simulink model "WPT_dc_source"  (R2022b)
settings: Solver=VariableStepAuto  StartTime=0.0  StopTime=10.0  RelTol=1e-3
libraries: spsMosfetLib x8, spsSeriesRLCBranchLib x6, spsVoltageMeasurementLib x6, spsDiodeLib x4, spsDCVoltageSourceLib x2, spsMutualInductanceLib x2, sps_lib x2
settings Model: Creator=SIDDHARTH  LastModifiedBy=SIDDHARTH

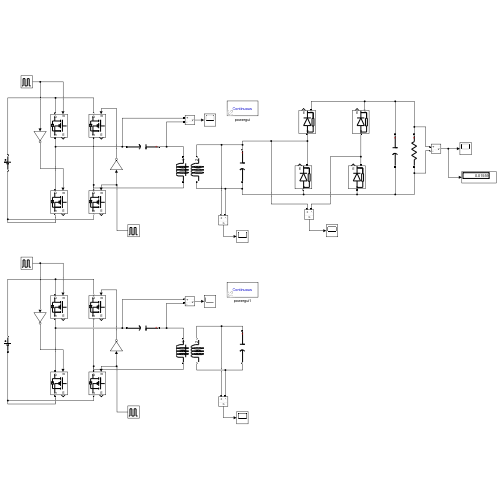
[thumbnail: Simulink's stored preview of the top-level diagram]
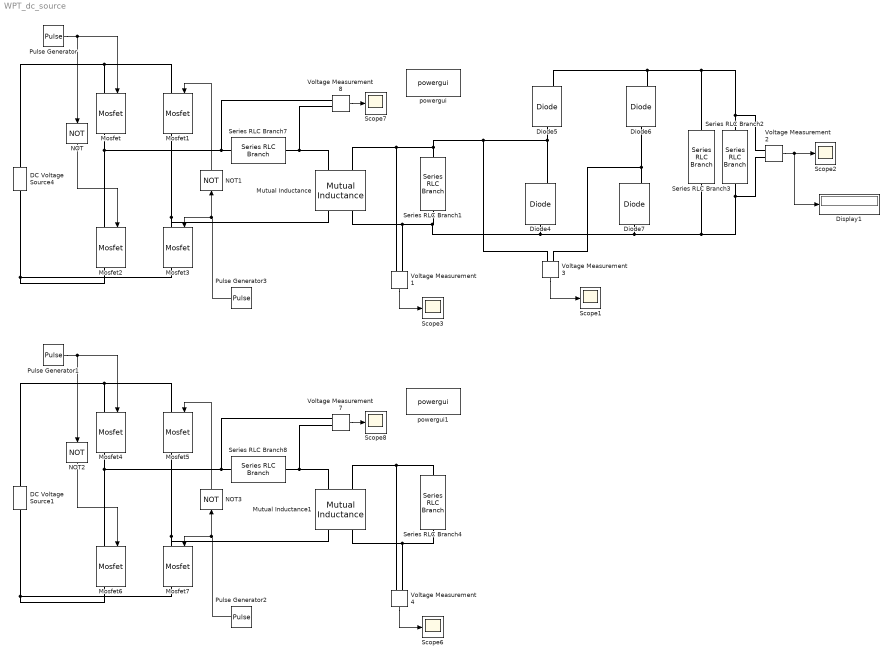
== system WPT_dc_source ==
  DC Voltage Source1 : spsDCVoltageSourceLib/DC Voltage Source  Amplitude=24  Measurements=None
  DC Voltage Source4 : spsDCVoltageSourceLib/DC Voltage Source  Amplitude=24  Measurements=None
  Diode4 : spsDiodeLib/Diode  Ron=0.001  Lon=0  Vf=0.7  IC=0  UseSnubber=0  Rs=500  Cs=250e-9  Measurements=on
  Diode5 : spsDiodeLib/Diode  Ron=0.001  Lon=0  Vf=0.8  IC=0  UseSnubber=0  Rs=500  Cs=250e-9  Measurements=on
  Diode6 : spsDiodeLib/Diode  Ron=0.001  Lon=0  Vf=0.7  IC=0  UseSnubber=0  Rs=500  Cs=250e-9  Measurements=on
  Diode7 : spsDiodeLib/Diode  Ron=0.001  Lon=0  Vf=0.7  IC=0  UseSnubber=0  Rs=500  Cs=250e-9  Measurements=on
  Display1 : Display
  Mosfet{,1..7} (8 alike) : spsMosfetLib/Mosfet  Ron=0.1  Lon=0  Rd=0.01  Vfd=0  IC=0  Rs=1e5  Cs=inf  Measurements=on
  Mutual Inductance : spsMutualInductanceLib/Mutual Inductance  LConnTagsString=a|b  RConnTagsString=A|B  TypeOfMutual=Two or three windings with equal mutual terms  NumberOfWindings=2  SelfImpedance1=[1e-2 1/(4*pi*pi*20000*(100e-6))]  SelfImpedance2=[1e-2 1/(4*pi*pi*20000*(100e-6))]  ThreeWindings=off  SelfImpedance3=[ 1.1 1.1e-03]  MutualImpedance=[0.9e-2 1.1207e-04]  InductanceMatrix="[1.0 0.9  0.9 ;  0.9 1.0  0.9;  0.9 0.9 1.0 ] * 1e-3"  ResistanceMatrix="[1.0 0.9  0.9 ;  0.9 1.0  0.9;  0.9 0.9 1.0 ]"  Measurements=Winding voltages
      settings: LibrarySourceBlock=sps_lib/Passives/Mutual Inductance
  Mutual Inductance1 : spsMutualInductanceLib/Mutual Inductance  LConnTagsString=a|b  RConnTagsString=A|B  TypeOfMutual=Two or three windings with equal mutual terms  NumberOfWindings=2  SelfImpedance1=[ 1.6054e-04 1/(4*pi*pi*20000*(100e-6))]  SelfImpedance2=[ 1.6054e-04 1/(4*pi*pi*20000*(100e-6))]  ThreeWindings=off  SelfImpedance3=[ 1.1 1.1e-03]  MutualImpedance=[ 1.6e-04 0.0099]  InductanceMatrix="[1.0 0.9  0.9 ;  0.9 1.0  0.9;  0.9 0.9 1.0 ] * 1e-3"  ResistanceMatrix="[1.0 0.9  0.9 ;  0.9 1.0  0.9;  0.9 0.9 1.0 ]"  Measurements=Winding voltages
      settings: LibrarySourceBlock=sps_lib/Passives/Mutual Inductance
  NOT{,1..3} (4 alike) : Logic  Operator=NOT  IconShape=distinctive  AllPortsSameDT=off  OutDataTypeStr=boolean
  Pulse Generator{,1..3} (4 alike) : DiscretePulseGenerator  PulseType=Time based  Period=1/20000  PulseWidth=75
  Scope{1..3,6..8} (6 alike) : Scope
  Series RLC Branch{1,4,7..8} (4 alike) : spsSeriesRLCBranchLib/Series RLC Branch  LConnTagsString=__new0  RConnTagsString=__new0  BranchType=C  Resistance=10  Inductance=1.02  SetiL0=off  InitialCurrent=0  Capacitance=100e-6  Setx0=off  InitialVoltage=0  Measurements=None
  Series RLC Branch2 : spsSeriesRLCBranchLib/Series RLC Branch  LConnTagsString=__new0  RConnTagsString=__new0  BranchType=R  Resistance=100000  Inductance=1e-3  SetiL0=off  InitialCurrent=0  Capacitance=1e-6  Setx0=off  InitialVoltage=0  Measurements=None
  Series RLC Branch3 : spsSeriesRLCBranchLib/Series RLC Branch  LConnTagsString=__new0  RConnTagsString=__new0  BranchType=C  Resistance=1  Inductance=1e-3  SetiL0=off  InitialCurrent=0  Capacitance=100e-6  Setx0=off  InitialVoltage=0  Measurements=Branch voltage
  Voltage Measurement{1..4,7..8} (6 alike) : spsVoltageMeasurementLib/Voltage Measurement  PhasorSimulation=off  OutputType=Complex  PSBequivalent=0
  powergui : sps_lib/powergui  Priority=1  SimulationMode=Continuous  SampleTime=50e-6  frequency=60  Iterations=50  frequencyindice=0  Pbase=100e6  ErrMax=1e-4  UnitsV=kV  UnitsW=MW  buscounter=0  FunctionMessages=off  echomessages=off  EnableUseOfTLC=off  CurrentSourceSwitches=off  DisableSnubberDevices=off  DisableRonSwitches=off  DisableVfSwitches=off  DisplayEquations=off  AutomaticDiscreteSolvers=off  SolverType=Tustin/Backward Euler (TBE)  Interpol=off  ExternalGateDelay=off  methode=off  Ts=100  x0status=blocks  SPID=on  SwTol=0  HookPort=off  NonlinearTolerance=1e-4  nMaxIteration=100  ContinueOnMaxIteration=off  RestoreLinks=warning  ResistiveCurrentMeasurement=off  Frange=[0:2:500]  Ylog=off  Xlog=on  ShowGrid=off  save=off  variable=ZData  structure=0  ZoomFFT=off  StartTime=0.0  cycles=1  DisplayStyle=1  fundamental=60  FreqAxis=off  MaxFrequency=1000  frequencyindicesteady=1  RmsSteady=1  display=off
  powergui1 : sps_lib/powergui  Priority=1  SimulationMode=Continuous  SampleTime=50e-6  frequency=60  Iterations=50  frequencyindice=0  Pbase=100e6  ErrMax=1e-4  UnitsV=kV  UnitsW=MW  buscounter=0  FunctionMessages=off  echomessages=off  EnableUseOfTLC=off  CurrentSourceSwitches=off  DisableSnubberDevices=off  DisableRonSwitches=off  DisableVfSwitches=off  DisplayEquations=off  AutomaticDiscreteSolvers=off  SolverType=Tustin/Backward Euler (TBE)  Interpol=off  ExternalGateDelay=off  methode=off  Ts=100  x0status=blocks  SPID=on  SwTol=0  HookPort=off  NonlinearTolerance=1e-4  nMaxIteration=100  ContinueOnMaxIteration=off  RestoreLinks=warning  ResistiveCurrentMeasurement=off  Frange=[0:2:500]  Ylog=off  Xlog=on  ShowGrid=off  save=off  variable=ZData  structure=0  ZoomFFT=off  StartTime=0.0  cycles=1  DisplayStyle=1  fundamental=60  FreqAxis=off  MaxFrequency=1000  frequencyindicesteady=1  RmsSteady=1  display=off
  wires:
  NOT/1 -> Mosfet2/1
  Pulse Generator3/1 -> NOT1/1, Mosfet3/1
  NOT1/1 -> Mosfet1/1
  Pulse Generator/1 -> Mosfet/1, NOT/1
  Voltage Measurement8/1 -> Scope7/1
  Voltage Measurement2/1 -> Display1/1, Scope2/1
  Voltage Measurement3/1 -> Scope1/1
  Voltage Measurement1/1 -> Scope3/1
  Pulse Generator2/1 -> NOT3/1, Mosfet7/1
  NOT2/1 -> Mosfet6/1
  NOT3/1 -> Mosfet5/1
  Voltage Measurement4/1 -> Scope6/1
  Pulse Generator1/1 -> Mosfet4/1, NOT2/1
  Voltage Measurement7/1 -> Scope8/1
  connections:
  Series RLC Branch7/LConn1 -- Mutual Inductance/LConn1 -- Voltage Measurement8/LConn2
  Mosfet/RConn1 -- Voltage Measurement8/LConn1 -- Series RLC Branch7/RConn1 -- Mosfet2/LConn1
  Mosfet3/RConn1 -- DC Voltage Source4/LConn1 -- Mosfet2/RConn1
  Mosfet1/RConn1 -- Mutual Inductance/RConn1 -- Mosfet3/LConn1
  Mosfet/LConn1 -- Mosfet1/LConn1 -- DC Voltage Source4/RConn1
  Voltage Measurement3/LConn1 -- Voltage Measurement1/LConn1 -- Mutual Inductance/LConn2 -- Series RLC Branch1/LConn1 -- Diode5/LConn1 -- Diode4/RConn1
  Voltage Measurement2/LConn2 -- Series RLC Branch2/RConn1 -- Series RLC Branch3/RConn1 -- Diode7/LConn1 -- Series RLC Branch1/RConn1 -- Voltage Measurement1/LConn2 -- Mutual Inductance/RConn2 -- Diode4/LConn1
  Diode6/LConn1 -- Voltage Measurement3/LConn2 -- Diode7/RConn1
  Series RLC Branch2/LConn1 -- Voltage Measurement2/LConn1 -- Series RLC Branch3/LConn1 -- Diode6/RConn1 -- Diode5/RConn1
  Mutual Inductance1/RConn2 -- Voltage Measurement4/LConn2 -- Series RLC Branch4/RConn1
  Mosfet7/LConn1 -- Mosfet5/RConn1 -- Mutual Inductance1/RConn1
  Mutual Inductance1/LConn2 -- Voltage Measurement4/LConn1 -- Series RLC Branch4/LConn1
  Series RLC Branch8/LConn1 -- Mutual Inductance1/LConn1 -- Voltage Measurement7/LConn2
  Mosfet7/RConn1 -- DC Voltage Source1/LConn1 -- Mosfet6/RConn1
  Mosfet4/RConn1 -- Voltage Measurement7/LConn1 -- Series RLC Branch8/RConn1 -- Mosfet6/LConn1
  Mosfet4/LConn1 -- Mosfet5/LConn1 -- DC Voltage Source1/RConn1
